simulink model "phase1"  (R2018b)
settings: Solver=VariableStepAuto  StartTime=0.0  StopTime=10  RelTol=1e-5
values from neighbouring files (symbols this model uses):
  b = 0.2    [SC_propoj.m]
  g = 9.8    [SC_propoj.m]
  I = 0.00651    [SC_propoj.m]
  Kg = 3.7    [SC_propoj.m]
  Km = 0.00767    [SC_propoj.m]
  l = 20    [SC_propoj.m]
  m = 0.210    (= 0.21)    [SC_propoj.m]
  M = 0.455    [SC_propoj.m]
  R = 2.6    [SC_propoj.m]
  r = 0.00635    [SC_propoj.m]
libraries: simulink_extras x2
settings Model: Creator=N.T  LastModifiedBy=N.T

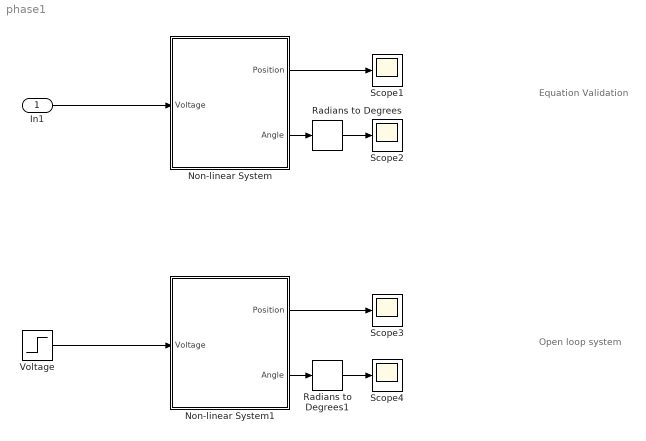
== system phase1 ==
  note: Equation Validation
  note: Open loop system
  In1 : Inport
  Non-linear System : Subsystem
  Non-linear System1 : Subsystem
  Radians to Degrees : simulink_extras/Transformations/Radians to Degrees
  Radians to Degrees1 : simulink_extras/Transformations/Radians to Degrees
  Scope{1..4} (4 alike) : Scope
  Voltage : Step  Time=0  Before=1  SampleTime=0
  wires:
  In1/1 -> Non-linear System/1(Voltage)
  Non-linear System1/1(Position) -> Scope3/1
  Non-linear System1/2(Angle) -> Radians to Degrees1/1
  Non-linear System/2(Angle) -> Radians to Degrees/1
  Non-linear System/1(Position) -> Scope1/1
  Radians to Degrees/1 -> Scope2/1
  Radians to Degrees1/1 -> Scope4/1
  Voltage/1 -> Non-linear System1/1(Voltage)

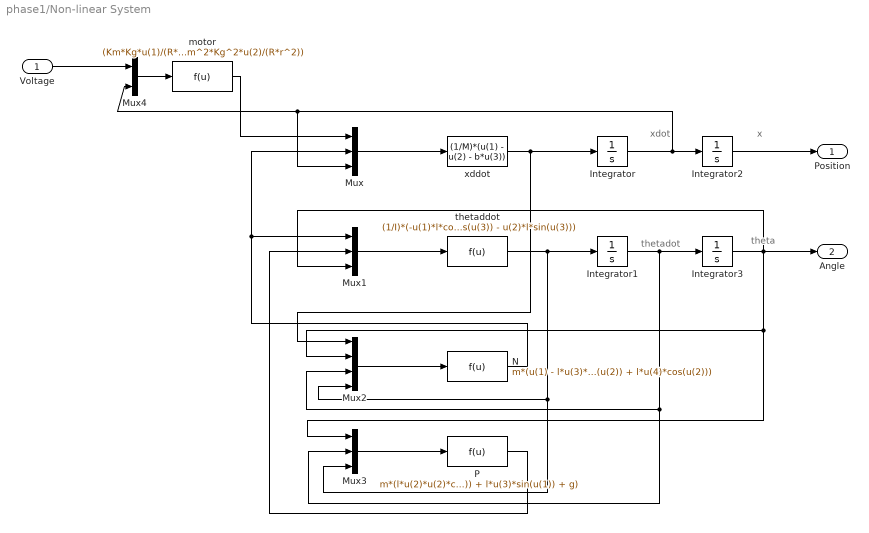
== system phase1/Non-linear System ==
  note: x
  note: thetadot
  note: xdot
  note: theta
  Voltage : Inport
  Integrator : Integrator  ContinuousStateAttributes='xdot'
  Integrator1 : Integrator  ContinuousStateAttributes='thetadot'
  Integrator2 : Integrator  ContinuousStateAttributes='x'
  Integrator3 : Integrator  InitialCondition=pi/2  ContinuousStateAttributes='theta'
  Mux : Mux  Inputs=3
  Mux1 : Mux  Inputs=3
  Mux2 : Mux
  Mux3 : Mux  Inputs=3
  Mux4 : Mux  Inputs=2
  N : Fcn  Expr=m*(u(1) - l*u(3)*u(3)*sin(u(2)) + l*u(4)*cos(u(2)))
  P : Fcn  Expr=m*(l*u(2)*u(2)*cos(u(1)) + l*u(3)*sin(u(1)) + g)
  motor : Fcn  Expr=(Km*Kg*u(1)/(R*r))-(Km^2*Kg^2*u(2)/(R*r^2))
  thetaddot : Fcn  Expr=(1/I)*(-u(1)*l*cos(u(3)) - u(2)*l*sin(u(3)))
  xddot : Fcn  Expr=(1/M)*(u(1) - u(2) - b*u(3))
  Position : Outport
  Angle : Outport  Port=2
  wires:
  Voltage/1 -> Mux4/1
  Mux4/1 -> motor/1
  thetaddot/1 -> Mux2/4, Mux3/3, Integrator1/1
  Mux2/1 -> N/1
  N/1 -> Mux1/1, Mux/2
  Integrator/1 -> Mux4/2, Mux/3, Integrator2/1
  Mux1/1 -> thetaddot/1
  Mux3/1 -> P/1
  xddot/1 -> Integrator/1, Mux2/1
  Integrator3/1 -> Mux3/1, Mux2/2, Angle/1, Mux1/3
  P/1 -> Mux1/2
  Integrator2/1 -> Position/1
  Mux/1 -> xddot/1
  Integrator1/1 -> Mux3/2, Mux2/3, Integrator3/1
  motor/1 -> Mux/1

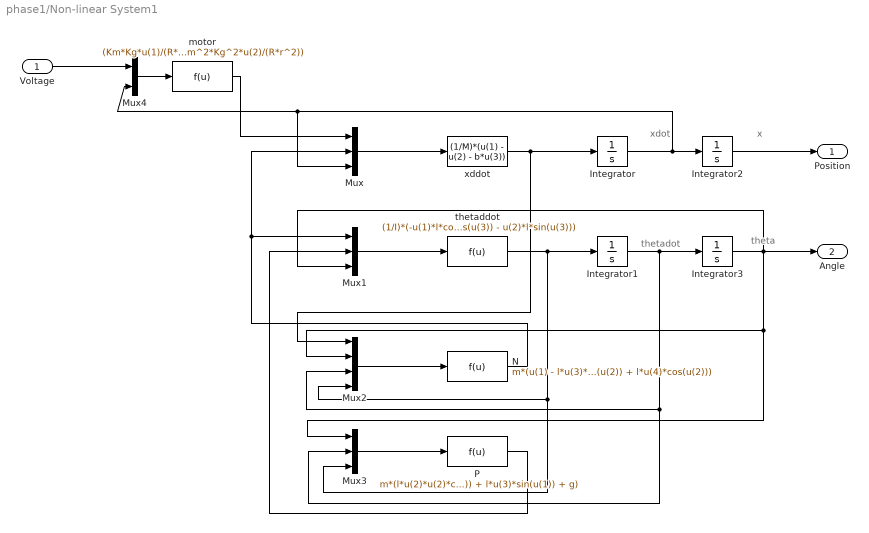
== system phase1/Non-linear System1 ==
  note: x
  note: thetadot
  note: xdot
  note: theta
  Voltage : Inport
  Integrator : Integrator  ContinuousStateAttributes='xdot'
  Integrator1 : Integrator  ContinuousStateAttributes='thetadot'
  Integrator2 : Integrator  ContinuousStateAttributes='x'
  Integrator3 : Integrator  InitialCondition=pi/2  ContinuousStateAttributes='theta'
  Mux : Mux  Inputs=3
  Mux1 : Mux  Inputs=3
  Mux2 : Mux
  Mux3 : Mux  Inputs=3
  Mux4 : Mux  Inputs=2
  N : Fcn  Expr=m*(u(1) - l*u(3)*u(3)*sin(u(2)) + l*u(4)*cos(u(2)))
  P : Fcn  Expr=m*(l*u(2)*u(2)*cos(u(1)) + l*u(3)*sin(u(1)) + g)
  motor : Fcn  Expr=(Km*Kg*u(1)/(R*r))-(Km^2*Kg^2*u(2)/(R*r^2))
  thetaddot : Fcn  Expr=(1/I)*(-u(1)*l*cos(u(3)) - u(2)*l*sin(u(3)))
  xddot : Fcn  Expr=(1/M)*(u(1) - u(2) - b*u(3))
  Position : Outport
  Angle : Outport  Port=2
  wires:
  Voltage/1 -> Mux4/1
  Mux4/1 -> motor/1
  thetaddot/1 -> Mux2/4, Mux3/3, Integrator1/1
  Mux2/1 -> N/1
  N/1 -> Mux1/1, Mux/2
  Integrator/1 -> Mux4/2, Mux/3, Integrator2/1
  Mux1/1 -> thetaddot/1
  Mux3/1 -> P/1
  xddot/1 -> Integrator/1, Mux2/1
  Integrator3/1 -> Mux3/1, Mux2/2, Angle/1, Mux1/3
  P/1 -> Mux1/2
  Integrator2/1 -> Position/1
  Mux/1 -> xddot/1
  Integrator1/1 -> Mux3/2, Mux2/3, Integrator3/1
  motor/1 -> Mux/1
